simulink model "CM640A_MotAg1Meas"  (R2013b)
settings: Solver=FixedStepDiscrete  SolverMode=SingleTasking  StartTime=0.0  StopTime=1  FixedStep=0.0000625  RelTol=1e-3
undefined symbols (not defined in the file): ARCHGLBPRM_2PI_ULS_F32, COEFFTBLELMSIZE_CNT_U08, COEFFTBLSIZE_CNT_U08, CORRNTBLAGSTEPSIZE_MATRAD_F32, CORRNTBLSIDXOFFS_CNT_U16, CORRNTBLSIZE_CNT_U16, CORRNTBLSIZEMASK_CNT_U08, MOTAG1OFFS_MOTREV_U0P16, MotAg1PrtclFlt, MOTAG1PRTCLFLTFAILSTEP_CNT_U16, MOTAG1PRTCLFLTPASSSTEP_CNT_U16, MOTAGDELTAPERCORRNPT_CNT_U16, MOTAGIDXMASK_CNT_U16, MotCtrlMotAg1ErrReg, NtcSts1, sigbuilder_block, SNSRAGMASK_CNT_U32, SNSRERRMASK_CNT_U32, SNSRERRNTCMASK_CNT_U08, SNSRVLTGFLTMASK_CNT_U32, SPIPARMASK_CNT_U32
libraries: simulink x28, FloatToFixd x1, NxtrMax x1, NxtrLim x1
(part 2 of 4)

== system CM640A_MotAg1Meas/MotAg1Meas/MotAg1MeasPer2/Process ErrorReg and DieRevCtr ==
  MotAg1ErrReg : Inport  OutDataTypeStr=uint32
  CopyRight2 : Subsystem  Description=|  mask(Copyright Information){none=on}
      | Copyright info block.                                               
      |                                                                     
      | Place copyright information at the top of every subsystem in design.
      mask prompts: none "No parameters"
      mask help: Place copyright information at the top of every subsystem in design.
      mask Display:
      | NxtrConf = 'Nexteer Confidential';
      | 
      | sys = bdroot; %handle for the current model ("system")
      | first = get_param(sys,'Created');
      | first = first(end-3:end);  %year is last four digits
      | 
      | last = get_param(sys,'LastModifiedDate');
      | if isempty(last)
      |     last = datestr(now,'yyyy');
      | else
      |     last = last(end-3:end);
      | end
      | 
      | if strcmp(first,last)
      |     fprintf('%s -- Copyright %s Nexteer',NxtrConf,first)
      | else
      |     fprintf('%s -- %s%s- %s Nexteer',NxtrConf,char(169),first,last)
      | end
  Process MotAg1RawErr : Subsystem  RequirementInfo={} %GIDa_05fef35d_e67f_443b_a4d0_6048385f8050
  MotAg1Err : Outport  OutDataTypeStr=uint8
  MotAg1ErrParFltCnt : Outport  Port=2
  wires:
  MotAg1ErrReg/1 -> Process MotAg1RawErr/1(MotAg1ErrReg)
  Process MotAg1RawErr/1(MotAg1ErrParFltCnt) -> MotAg1ErrParFltCnt/1
  Process MotAg1RawErr/2(MotAg1Err) -> MotAg1Err/1

== system CM640A_MotAg1Meas/MotAg1Meas/MotAg1MeasInit1/Compute Correction Table/CopyRight2 ==

== system CM640A_MotAg1Meas/MotAg1Meas/MotAg1MeasInit1/Compute Correction Table/MotAg1CorrnTbl_GetErrorStatus ==
  note: 0 simulated for modeling purposes,
      | actual value returned by NVM.  Non-zero return indicates
      | failure in storage/retrievial of NVM.
  Constant : Constant  Value=0
  CopyRight2 : Subsystem  Description=|  mask(Copyright Information){none=on}
      | Copyright info block.                                               
      |                                                                     
      | Place copyright information at the top of every subsystem in design.
      mask prompts: none "No parameters"
      mask help: Place copyright information at the top of every subsystem in design.
      mask Display:
      | NxtrConf = 'Nexteer Confidential';
      | 
      | sys = bdroot; %handle for the current model ("system")
      | first = get_param(sys,'Created');
      | first = first(end-3:end);  %year is last four digits
      | 
      | last = get_param(sys,'LastModifiedDate');
      | if isempty(last)
      |     last = datestr(now,'yyyy');
      | else
      |     last = last(end-3:end);
      | end
      | 
      | if strcmp(first,last)
      |     fprintf('%s -- Copyright %s Nexteer',NxtrConf,first)
      | else
      |     fprintf('%s -- %s%s- %s Nexteer',NxtrConf,char(169),first,last)
      | end
  RequestResultPtr : Outport
  wires:
  Constant/1 -> RequestResultPtr/1

== system CM640A_MotAg1Meas/MotAg1Meas/MotAg1MeasInit1/Compute Correction Table/NVM NOK ==
  note: In the event of a NVM failure
      | set the correction table to 0
  Action Port : ActionPort  ActionType=else
  Constant1 : Constant  Value=CORRNTBLSIZE_CNT_U16
  CopyRight2 : Subsystem  Description=|  mask(Copyright Information){none=on}
      | Copyright info block.                                               
      |                                                                     
      | Place copyright information at the top of every subsystem in design.
      mask prompts: none "No parameters"
      mask help: Place copyright information at the top of every subsystem in design.
      mask Display:
      | NxtrConf = 'Nexteer Confidential';
      | 
      | sys = bdroot; %handle for the current model ("system")
      | first = get_param(sys,'Created');
      | first = first(end-3:end);  %year is last four digits
      | 
      | last = get_param(sys,'LastModifiedDate');
      | if isempty(last)
      |     last = datestr(now,'yyyy');
      | else
      |     last = last(end-3:end);
      | end
      | 
      | if strcmp(first,last)
      |     fprintf('%s -- Copyright %s Nexteer',NxtrConf,first)
      | else
      |     fprintf('%s -- %s%s- %s Nexteer',NxtrConf,char(169),first,last)
      | end
  Zero out correction table : Subsystem  TreatAsAtomicUnit=on
  wires:
  Constant1/1 -> Zero out correction table/1(N)

== system CM640A_MotAg1Meas/MotAg1Meas/MotAg1MeasInit1/Compute Correction Table/NVM Ok ==
  Action Port : ActionPort  ActionType=then
  Calculate Correction Table : Subsystem  Priority=100  TreatAsAtomicUnit=on
      settings: AttributesFormatString=|
      | Priority:
      | %<Priority>
  Configure Coefficients : Subsystem  Priority=10  TreatAsAtomicUnit=on
      settings: AttributesFormatString=|
      | Priority:
      | %<Priority>
  CopyRight2 : Subsystem  Description=|  mask(Copyright Information){none=on}
      | Copyright info block.                                               
      |                                                                     
      | Place copyright information at the top of every subsystem in design.
      mask prompts: none "No parameters"
      mask help: Place copyright information at the top of every subsystem in design.
      mask Display:
      | NxtrConf = 'Nexteer Confidential';
      | 
      | sys = bdroot; %handle for the current model ("system")
      | first = get_param(sys,'Created');
      | first = first(end-3:end);  %year is last four digits
      | 
      | last = get_param(sys,'LastModifiedDate');
      | if isempty(last)
      |     last = datestr(now,'yyyy');
      | else
      |     last = last(end-3:end);
      | end
      | 
      | if strcmp(first,last)
      |     fprintf('%s -- Copyright %s Nexteer',NxtrConf,first)
      | else
      |     fprintf('%s -- %s%s- %s Nexteer',NxtrConf,char(169),first,last)
      | end

== system CM640A_MotAg1Meas/MotAg1Meas/MotAg1MeasInit1/Initialize CSIH RAM1/CopyRight2 ==

== system CM640A_MotAg1Meas/MotAg1Meas/MotAg1MeasPer1/Compensate MechMtrPos/CopyRight1 ==

== system CM640A_MotAg1Meas/MotAg1Meas/MotAg1MeasPer1/Process MotAg1 Angle/CopyRight2 ==

== system CM640A_MotAg1Meas/MotAg1Meas/MotAg1MeasPer1/Process MotAg1 Angle/Process MotAg1Raw ==
  RxMtrPosReg_Cnt_u32 : Inport  OutDataTypeStr=uint32
  CopyRight2 : Subsystem  Description=|  mask(Copyright Information){none=on}
      | Copyright info block.                                               
      |                                                                     
      | Place copyright information at the top of every subsystem in design.
      mask prompts: none "No parameters"
      mask help: Place copyright information at the top of every subsystem in design.
      mask Display:
      | NxtrConf = 'Nexteer Confidential';
      | 
      | sys = bdroot; %handle for the current model ("system")
      | first = get_param(sys,'Created');
      | first = first(end-3:end);  %year is last four digits
      | 
      | last = get_param(sys,'LastModifiedDate');
      | if isempty(last)
      |     last = datestr(now,'yyyy');
      | else
      |     last = last(end-3:end);
      | end
      | 
      | if strcmp(first,last)
      |     fprintf('%s -- Copyright %s Nexteer',NxtrConf,first)
      | else
      |     fprintf('%s -- %s%s- %s Nexteer',NxtrConf,char(169),first,last)
      | end
  MotAg Message Parity Monitoring : Subsystem  RequirementInfo="{'linktype_rmi_doors' '0000cf48 (/ESG Group/FDD Module Requirements/EA4 Specific/CM640A_MotAg1Meas)' '#CM640A_93' 'true' 'REQ:  CM640A_93' '' } %GIDa_0575b366_3fb8_4b54_8653_e88c552f3ea4"  TreatAsAtomicUnit=on
  Raw Mecl Mot Ag Processing : Subsystem  RequirementInfo="{'linktype_rmi_doors' '0000cf48 (/ESG Group/FDD Module Requirements/EA4 Specific/CM640A_MotAg1Meas)' '#CM640A_84' 'true' 'REQ:  CM640A_84' '' } %GIDa_bdb55e65_3f35_4b3c_b59f_3789084d0974"  TreatAsAtomicUnit=on
  Undervoltage Bit Monitoring : Subsystem  RequirementInfo="{'linktype_rmi_doors' '0000cf48 (/ESG Group/FDD Module Requirements/EA4 Specific/CM640A_MotAg1Meas)' '#CM640A_86' 'true' 'REQ:  CM640A_86' '' } %GIDa_7bdb6e2d_fd76_45a7_a9c7_b8b57ac688de"  TreatAsAtomicUnit=on
  MotAg1VltgFlt : Outport
  MotAg1ParFlt : Outport  Port=2
  MotAg1RawMecl : Outport  Port=3
  wires:
  RxMtrPosReg_Cnt_u32/1 -> Raw Mecl Mot Ag Processing/1(RxMtrPosReg_Cnt_u32), MotAg Message Parity Monitoring/1(RxMtrPosReg_Cnt_u32), Undervoltage Bit Monitoring/1(RxMtrPosReg_Cnt_u32)
  Raw Mecl Mot Ag Processing/1(MotAg1RawMecl) -> MotAg1RawMecl/1
  Undervoltage Bit Monitoring/1(MotAg1VltgFlt) -> MotAg1VltgFlt/1
  MotAg Message Parity Monitoring/1(MotAg1ParFlt) -> MotAg1ParFlt/1

== system CM640A_MotAg1Meas/MotAg1Meas/MotAg1MeasPer1/Process MotAg1 Angle/Protocol Present Handling ==
  Protocol Fault Present : Inport
  MotAg1RawMecl Input : Inport  Port=2
  CopyRight2 : Subsystem  Description=|  mask(Copyright Information){none=on}
      | Copyright info block.                                               
      |                                                                     
      | Place copyright information at the top of every subsystem in design.
      mask prompts: none "No parameters"
      mask help: Place copyright information at the top of every subsystem in design.
      mask Display:
      | NxtrConf = 'Nexteer Confidential';
      | 
      | sys = bdroot; %handle for the current model ("system")
      | first = get_param(sys,'Created');
      | first = first(end-3:end);  %year is last four digits
      | 
      | last = get_param(sys,'LastModifiedDate');
      | if isempty(last)
      |     last = datestr(now,'yyyy');
      | else
      |     last = last(end-3:end);
      | end
      | 
      | if strcmp(first,last)
      |     fprintf('%s -- Copyright %s Nexteer',NxtrConf,first)
      | else
      |     fprintf('%s -- %s%s- %s Nexteer',NxtrConf,char(169),first,last)
      | end
  If : If  IfExpression=u1 == 0
  "Invalid Polarity, Hold Last Value" : Subsystem  TreatAsAtomicUnit=on
  Merge : Merge  RequirementInfo={} %GIDa_c39e7a9a_c902_423e_a1fe_e344504ccac1
  Unit Delay3 : UnitDelay  SampleTime=-1  StateName=MotAg1RawMeclPrev  StateMustResolveToSignalObject=on
      settings: AttributesFormatString=|
      | State Variable:
      | %<StateName>
  Valid Polarity : Subsystem  TreatAsAtomicUnit=on
  MotAg1RawMecl : Outport
  wires:
  Unit Delay3/1 -> "Invalid Polarity, Hold Last Value"/1(In1)
  Merge/1 -> MotAg1RawMecl/1, Unit Delay3/1
  "Invalid Polarity, Hold Last Value"/1(Out1) -> Merge/2
  Valid Polarity/1(Out1) -> Merge/1
  If/2 -> "Invalid Polarity, Hold Last Value"/Action
  If/1 -> Valid Polarity/Action
  MotAg1RawMecl Input/1 -> Valid Polarity/1(In1)
  Protocol Fault Present/1 -> If/1

== system CM640A_MotAg1Meas/MotAg1Meas/MotAg1MeasPer2/MotAg1 Protocol Fault Operation/Atomic Subsystem ==
  NtcStInfo : Inport  OutDataTypeStr=uint8
  CopyRight2 : Subsystem  Description=|  mask(Copyright Information){none=on}
      | Copyright info block.                                               
      |                                                                     
      | Place copyright information at the top of every subsystem in design.
      mask prompts: none "No parameters"
      mask help: Place copyright information at the top of every subsystem in design.
      mask Display:
      | NxtrConf = 'Nexteer Confidential';
      | 
      | sys = bdroot; %handle for the current model ("system")
      | first = get_param(sys,'Created');
      | first = first(end-3:end);  %year is last four digits
      | 
      | last = get_param(sys,'LastModifiedDate');
      | if isempty(last)
      |     last = datestr(now,'yyyy');
      | else
      |     last = last(end-3:end);
      | end
      | 
      | if strcmp(first,last)
      |     fprintf('%s -- Copyright %s Nexteer',NxtrConf,first)
      | else
      |     fprintf('%s -- %s%s- %s Nexteer',NxtrConf,char(169),first,last)
      | end
  If : If
  Merge : Merge
  Merge1 : Merge
  N Step : Subsystem  RequirementInfo="{'linktype_rmi_doors' '0000cf48 (/ESG Group/FDD Module Requirements/EA4 Specific/CM640A_MotAg1Meas)' '#CM640A_31' 'true' 'REQ:  CM640A_31' '' } %GIDa_a1ed8da0_4c35_4cb0_a2c6_08587c652881"  TreatAsAtomicUnit=on
  P Step : Subsystem  TreatAsAtomicUnit=on
  NtcSts : Outport
  DebStep : Outport  Port=2  OutDataTypeStr=uint16
  wires:
  NtcStInfo/1 -> If/1
  If/1 -> P Step/Action
  If/2 -> N Step/Action
  Merge/1 -> DebStep/1
  P Step/1(NtcSts) -> Merge1/1
  N Step/1(NtcSts) -> Merge1/2
  Merge1/1 -> NtcSts/1
  P Step/2(DebStep) -> Merge/1
  N Step/2(DebStep) -> Merge/2

== system CM640A_MotAg1Meas/MotAg1Meas/MotAg1MeasPer2/MotAg1 Protocol Fault Operation/CopyRight2 ==

== system CM640A_MotAg1Meas/MotAg1Meas/MotAg1MeasPer2/MotAg1 Protocol Fault Operation/GetNtcQlfr ==
  NtcNr : Inport
  CopyRight2 : Subsystem  Description=|  mask(Copyright Information){none=on}
      | Copyright info block.                                               
      |                                                                     
      | Place copyright information at the top of every subsystem in design.
      mask prompts: none "No parameters"
      mask help: Place copyright information at the top of every subsystem in design.
      mask Display:
      | NxtrConf = 'Nexteer Confidential';
      | 
      | sys = bdroot; %handle for the current model ("system")
      | first = get_param(sys,'Created');
      | first = first(end-3:end);  %year is last four digits
      | 
      | last = get_param(sys,'LastModifiedDate');
      | if isempty(last)
      |     last = datestr(now,'yyyy');
      | else
      |     last = last(end-3:end);
      | end
      | 
      | if strcmp(first,last)
      |     fprintf('%s -- Copyright %s Nexteer',NxtrConf,first)
      | else
      |     fprintf('%s -- %s%s- %s Nexteer',NxtrConf,char(169),first,last)
      | end
  Data Store Read : DataStoreRead  DataStoreName=NtcQlfr
  Terminator : Terminator
  NtcQlfr : Outport
  wires:
  NtcNr/1 -> Terminator/1
  Data Store Read/1 -> NtcQlfr/1

== system CM640A_MotAg1Meas/MotAg1Meas/MotAg1MeasPer2/MotAg1 Protocol Fault Operation/SetNtcSts ==
  note: Note:
      |
      | - "ISO Fault Debounce Design" Simulink block intent to use here for Simulation purpose only. Do not Code this block
  NtcNr : Inport
  NtcStInfo : Inport  Port=2
  NtcSts : Inport  Port=3  OutDataTypeStr=Enum: NtcSts1
  DebStep : Inport  Port=4
  CopyRight2 : Subsystem  Description=|  mask(Copyright Information){none=on}
      | Copyright info block.                                               
      |                                                                     
      | Place copyright information at the top of every subsystem in design.
      mask prompts: none "No parameters"
      mask help: Place copyright information at the top of every subsystem in design.
      mask Display:
      | NxtrConf = 'Nexteer Confidential';
      | 
      | sys = bdroot; %handle for the current model ("system")
      | first = get_param(sys,'Created');
      | first = first(end-3:end);  %year is last four digits
      | 
      | last = get_param(sys,'LastModifiedDate');
      | if isempty(last)
      |     last = datestr(now,'yyyy');
      | else
      |     last = last(end-3:end);
      | end
      | 
      | if strcmp(first,last)
      |     fprintf('%s -- Copyright %s Nexteer',NxtrConf,first)
      | else
      |     fprintf('%s -- %s%s- %s Nexteer',NxtrConf,char(169),first,last)
      | end
  Data Store Write : DataStoreWrite  DataStoreName=NtcQlfr
  Data Type Conversion1 : DataTypeConversion  OutDataTypeStr=uint8
  Ground : Ground
  ISO Fault Debounce Design : Stateflow chart  TreatAsAtomicUnit=on
      settings: AttributesFormatString=|
      | Simulation Purpose Only.
      | Do Not Code this block
      | Diagnostic Manager Owns this requirement
  Scope1 : Scope  NumInputPorts=4
      settings: YMin=-5~-5~-5~-5  YMax=5~5~5~5  SaveName=ScopeData5
  Terminator : Terminator
  Terminator1 : Terminator
  wires:
  NtcStInfo/1 -> Scope1/4, Terminator1/1
  NtcNr/1 -> Terminator/1
  NtcSts/1 -> Data Type Conversion1/1
  DebStep/1 -> ISO Fault Debounce Design/2(DebStep), Scope1/2
  ISO Fault Debounce Design/1(Qualifier) -> Scope1/3, Data Store Write/1
  Ground/1 -> ISO Fault Debounce Design/3(SvcClr)
  Data Type Conversion1/1 -> ISO Fault Debounce Design/1(NtcSts), Scope1/1

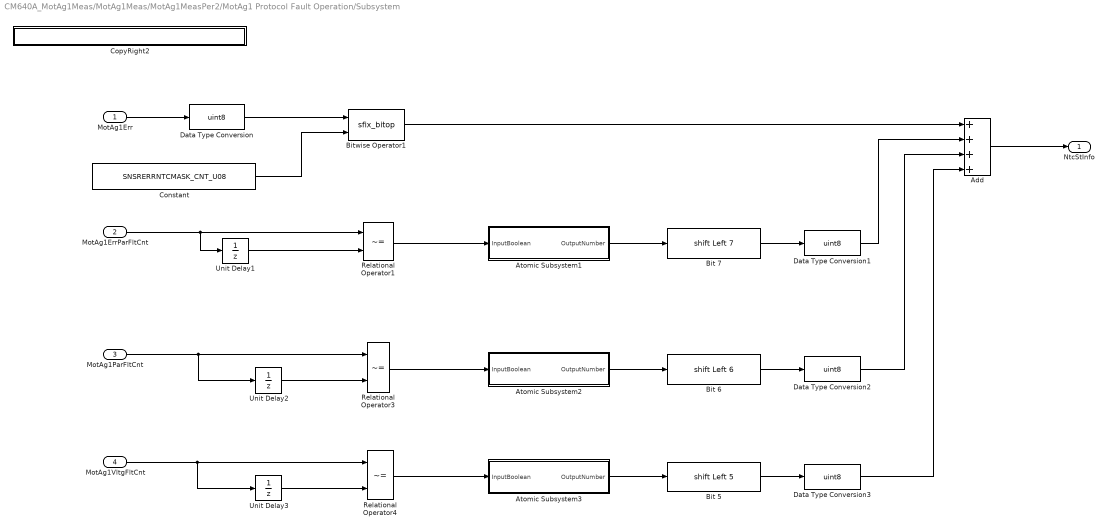
== system CM640A_MotAg1Meas/MotAg1Meas/MotAg1MeasPer2/MotAg1 Protocol Fault Operation/Subsystem ==
  MotAg1Err : Inport  RequirementInfo={} %GIDa_6edd1ae9_9c74_4544_bf40_7d9417b836a7
  MotAg1ErrParFltCnt : Inport  Port=2
  MotAg1ParFltCnt : Inport  Port=3
  MotAg1VltgFltCnt : Inport  Port=4
  Add : Sum  Inputs=++++
  Atomic Subsystem1 : Subsystem  TreatAsAtomicUnit=on
  Atomic Subsystem2 : Subsystem  TreatAsAtomicUnit=on
  Atomic Subsystem3 : Subsystem  TreatAsAtomicUnit=on
  Bit 5 : ArithShift  RequirementInfo="{'linktype_rmi_doors' '0000cf48 (/ESG Group/FDD Module Requirements/EA4 Specific/CM640A_MotAg1Meas)' '#CM640A_28' 'true' 'REQ:  CM640A_28' '' } %GIDa_baaec4dd_391c_4963_979e_8a787ae9f4f7"  BitShiftNumber=5  BitShiftDirection=Left
  Bit 6 : ArithShift  RequirementInfo="{'linktype_rmi_doors' '0000cf48 (/ESG Group/FDD Module Requirements/EA4 Specific/CM640A_MotAg1Meas)' '#CM640A_101' 'true' 'REQ:  CM640A_101' '' } %GIDa_688756ca_05b1_4787_ba54_8f8dae8f5212"  BitShiftNumber=6  BitShiftDirection=Left
  Bit 7 : ArithShift  RequirementInfo="{'linktype_rmi_doors' '0000cf48 (/ESG Group/FDD Module Requirements/EA4 Specific/CM640A_MotAg1Meas)' '#CM640A_102' 'true' 'REQ:  CM640A_102' '' } %GIDa_5f89c88f_2af9_4850_b51d_5320054dccdc"  BitShiftNumber=7  BitShiftDirection=Left
  Bitwise Operator1 : S-Function  RequirementInfo="{'linktype_rmi_doors' '0000cf48 (/ESG Group/FDD Module Requirements/EA4 Specific/CM640A_MotAg1Meas)' '#CM640A_91' 'true' 'REQ:  CM640A_91' '' ; 'linktype_rmi_doors' '0000cf48 (/ESG Group/FDD Module Requirements/EA4 Specific/CM640A_MotAg1Meas)' '#CM640A_98' 'true' 'REQ:  CM640A_98' '' ; 'linktype_rmi_doors' '0000cf48 (/ESG Group/FDD Module Requirements/EA4 Specific/CM640A_MotAg1Meas)' '#CM640A_99' 'true' 'REQ:  CM640A_99' '' ; 'linktype_rmi_doors' '0000cf48 (/ESG Group/FDD Module Requirements/EA4 Specific/CM640A_MotAg1Meas)' '#CM640A_100' 'true' 'REQ:  CM640A_100' '' } %GIDa_5c9d0cb2_6ffb_4aa7_875c_2abe2058166d"  FunctionName=sfix_bitop  Parameters=UseBitMask,NumInputPorts,BitMask,BitMaskRealWorld,logicop  EnableBusSupport=off  mask(Bitwise Operator){logicop=AND, UseBitMask=off, NumInputPorts=2, BitMask=SNSRERRNTCMASK_CNT_U08, BitMaskRealWorld=Stored Integer}
      mask prompts: logicop "Operator:"; UseBitMask "Use bit mask ..."; NumInputPorts "Number of input ports:"; BitMask "Bit Mask"; BitMaskRealWorld "Treat mask as:"
      mask help: Perform the specified bitwise operation on the inputs. The output data type should represent zero exactly.
      mask init:
      | str = '';
      | if UseBitMask
      |   [m,n] = size(BitMask);
      |   if ischar(BitMask)
      |     len = m;
      |     n = 1;
      |   else
      |     len = m * n;
      |   end
      |   internalBitMask = zeros(m,n);
      |   if isnumeric(BitMask)
      |     for i=1:len,
      |       internalBitMask(i) = BitMask(i);
      |     end
      |   elseif ischar(BitMask)
      |     for i=1:m,
      |       internalBitMask(i) = hex2dec(BitMask(i,:));
      |     end
      |   elseif iscell(BitMask)
      |     for i=1:len,
      |       if isnumeric( BitMask{i} )
      |         internalBitMask(i) = BitMask{i};
      |       elseif ischar( BitMask{i} )
      |         internalBitMask(i) = hex2dec(BitMask{i});
      |       else
      |         errordlg(['Data type is not supported at cell item ', num2str(i) ]);
      |       end
      |     end
      |   end
      |   BitMask = internalBitMask;
      |   for i=1:len
      |     if BitMask(i) > (2^52)-1
      |       error(DAStudio.message('Simulink:blocks:BitMaskWordLengthTooLarge')); 
      |     end
      |   end 
      |   if len == 1
      |      if BitMaskRealWorld == 1 || BitMask(1) < 0
      |        str=num2str(BitMask(1));
      |      else
      |        str=['0x',dec2hex(floor(BitMask(1)))];
      |      end
      |   else
      |      str='Masks';
      |   end
      | else
      |   BitMask = 0;
      |   str='';
      | end
      mask TypeOptions logicop: AND | OR | NAND | NOR | XOR | NOT
      mask Callback logicop: fixptdialog(gcbh)
      mask Callback UseBitMask: fixptdialog(gcbh)
      mask TypeOptions BitMaskRealWorld: Real World Value | Stored Integer
      mask Display: fprintf(['Bitwise\n',logicop,'\n',str])
  Constant : Constant  Value=SNSRERRNTCMASK_CNT_U08
  CopyRight2 : Subsystem  Description=|  mask(Copyright Information){none=on}
      | Copyright info block.                                               
      |                                                                     
      | Place copyright information at the top of every subsystem in design.
      mask prompts: none "No parameters"
      mask help: Place copyright information at the top of every subsystem in design.
      mask Display:
      | NxtrConf = 'Nexteer Confidential';
      | 
      | sys = bdroot; %handle for the current model ("system")
      | first = get_param(sys,'Created');
      | first = first(end-3:end);  %year is last four digits
      | 
      | last = get_param(sys,'LastModifiedDate');
      | if isempty(last)
      |     last = datestr(now,'yyyy');
      | else
      |     last = last(end-3:end);
      | end
      | 
      | if strcmp(first,last)
      |     fprintf('%s -- Copyright %s Nexteer',NxtrConf,first)
      | else
      |     fprintf('%s -- %s%s- %s Nexteer',NxtrConf,char(169),first,last)
      | end
  Data Type Conversion{,1..3} (4 alike) : DataTypeConversion  OutDataTypeStr=uint8
  Relational Operator1 : RelationalOperator  Operator=~=  OutDataTypeStr=boolean
  Relational Operator3 : RelationalOperator  Operator=~=  OutDataTypeStr=boolean
  Relational Operator4 : RelationalOperator  Operator=~=  OutDataTypeStr=boolean
  Unit Delay1 : UnitDelay  SampleTime=-1  StateName=MotAg1ErrParFltNtcStInfoCntPrev  StateMustResolveToSignalObject=on
      settings: AttributesFormatString=|
      | State Variable:
      | %<StateName>
  Unit Delay2 : UnitDelay  SampleTime=-1  StateName=MotAg1ParFltNtcStInfoCntPrev  StateMustResolveToSignalObject=on
      settings: AttributesFormatString=|
      | State Variable:
      | %<StateName>
  Unit Delay3 : UnitDelay  SampleTime=-1  StateName=MotAg1VltgFltNtcStInfoCntPrev  StateMustResolveToSignalObject=on
      settings: AttributesFormatString=|
      | State Variable:
      | %<StateName>
  NtcStInfo : Outport
  wires:
  Add/1 -> NtcStInfo/1
  Relational Operator3/1 -> Atomic Subsystem2/1(InputBoolean)
  MotAg1ParFltCnt/1 -> Unit Delay2/1, Relational Operator3/1
  Unit Delay1/1 -> Relational Operator1/2
  MotAg1ErrParFltCnt/1 -> Unit Delay1/1, Relational Operator1/1
  MotAg1Err/1 -> Data Type Conversion/1
  Data Type Conversion/1 -> Bitwise Operator1/1
  Relational Operator4/1 -> Atomic Subsystem3/1(InputBoolean)
  Unit Delay3/1 -> Relational Operator4/2
  MotAg1VltgFltCnt/1 -> Unit Delay3/1, Relational Operator4/1
  Bitwise Operator1/1 -> Add/1
  Unit Delay2/1 -> Relational Operator3/2
  Relational Operator1/1 -> Atomic Subsystem1/1(InputBoolean)
  Atomic Subsystem1/1(OutputNumber) -> Bit 7/1
  Atomic Subsystem2/1(OutputNumber) -> Bit 6/1
  Atomic Subsystem3/1(OutputNumber) -> Bit 5/1
  Data Type Conversion3/1 -> Add/4
  Data Type Conversion2/1 -> Add/3
  Data Type Conversion1/1 -> Add/2
  Bit 5/1 -> Data Type Conversion3/1
  Bit 6/1 -> Data Type Conversion2/1
  Bit 7/1 -> Data Type Conversion1/1
  Constant/1 -> Bitwise Operator1/2

== system CM640A_MotAg1Meas/MotAg1Meas/MotAg1MeasPer2/Process ErrorReg and DieRevCtr/CopyRight2 ==

== system CM640A_MotAg1Meas/MotAg1Meas/MotAg1MeasPer2/Process ErrorReg and DieRevCtr/Process MotAg1RawErr ==
  MotAg1ErrReg : Inport
  Chart1 : Stateflow chart  TreatAsAtomicUnit=on
  CopyRight2 : Subsystem  Description=|  mask(Copyright Information){none=on}
      | Copyright info block.                                               
      |                                                                     
      | Place copyright information at the top of every subsystem in design.
      mask prompts: none "No parameters"
      mask help: Place copyright information at the top of every subsystem in design.
      mask Display:
      | NxtrConf = 'Nexteer Confidential';
      | 
      | sys = bdroot; %handle for the current model ("system")
      | first = get_param(sys,'Created');
      | first = first(end-3:end);  %year is last four digits
      | 
      | last = get_param(sys,'LastModifiedDate');
      | if isempty(last)
      |     last = datestr(now,'yyyy');
      | else
      |     last = last(end-3:end);
      | end
      | 
      | if strcmp(first,last)
      |     fprintf('%s -- Copyright %s Nexteer',NxtrConf,first)
      | else
      |     fprintf('%s -- %s%s- %s Nexteer',NxtrConf,char(169),first,last)
      | end
  Data Type Conversion1 : DataTypeConversion  OutDataTypeStr=uint16
  If : If  IfExpression=u1 == 0
  "Invalid Polarity, Hold Last Value" : Subsystem  TreatAsAtomicUnit=on
  Merge : Merge
  Process MotAg1RawErr : Subsystem
  Unit Delay1 : UnitDelay  SampleTime=-1  StateName=MotAg1ErrParFltCntPrev  StateMustResolveToSignalObject=on
      settings: AttributesFormatString=|
      | State Variable:
      | %<StateName>
  Unit Delay3 : UnitDelay  SampleTime=-1  StateName=MotAg1ErrPrev  StateMustResolveToSignalObject=on
      settings: AttributesFormatString=|
      | State Variable:
      | %<StateName>
  Valid Polarity : Subsystem  TreatAsAtomicUnit=on
  MotAg1ErrParFltCnt : Outport
  MotAg1Err : Outport  Port=2  OutDataTypeStr=uint8
  wires:
  Process MotAg1RawErr/1(MotAg1ErrParFlt) -> If/1, Data Type Conversion1/1
  Unit Delay3/1 -> "Invalid Polarity, Hold Last Value"/1(In1)
  Merge/1 -> Unit Delay3/1, MotAg1Err/1
  MotAg1ErrReg/1 -> Process MotAg1RawErr/1(MotAg1ErrReg)
  "Invalid Polarity, Hold Last Value"/1(Out1) -> Merge/2
  Valid Polarity/1(Out1) -> Merge/1
  If/2 -> "Invalid Polarity, Hold Last Value"/Action
  If/1 -> Valid Polarity/Action
  Process MotAg1RawErr/2(MotAg1Err) -> Valid Polarity/1(In1)
  Data Type Conversion1/1 -> Chart1/1(Fault)
  Chart1/1(FaultCnt) -> MotAg1ErrParFltCnt/1, Unit Delay1/1
  Unit Delay1/1 -> Chart1/2(FaultCntPrev)

== system CM640A_MotAg1Meas/MotAg1Meas/MotAg1MeasInit1/Compute Correction Table/MotAg1CorrnTbl_GetErrorStatus/CopyRight2 ==

== system CM640A_MotAg1Meas/MotAg1Meas/MotAg1MeasInit1/Compute Correction Table/NVM NOK/CopyRight2 ==

== system CM640A_MotAg1Meas/MotAg1Meas/MotAg1MeasInit1/Compute Correction Table/NVM NOK/Zero out correction table ==
  N : Inport
  Assignment : Assignment  IndexMode=Zero-based  IndexOptions=Index vector (port)  Indices=1  OutputSizes=1
  CopyRight2 : Subsystem  Description=|  mask(Copyright Information){none=on}
      | Copyright info block.                                               
      |                                                                     
      | Place copyright information at the top of every subsystem in design.
      mask prompts: none "No parameters"
      mask help: Place copyright information at the top of every subsystem in design.
      mask Display:
      | NxtrConf = 'Nexteer Confidential';
      | 
      | sys = bdroot; %handle for the current model ("system")
      | first = get_param(sys,'Created');
      | first = first(end-3:end);  %year is last four digits
      | 
      | last = get_param(sys,'LastModifiedDate');
      | if isempty(last)
      |     last = datestr(now,'yyyy');
      | else
      |     last = last(end-3:end);
      | end
      | 
      | if strcmp(first,last)
      |     fprintf('%s -- Copyright %s Nexteer',NxtrConf,first)
      | else
      |     fprintf('%s -- %s%s- %s Nexteer',NxtrConf,char(169),first,last)
      | end
  Data Store Read : DataStoreRead  DataStoreName=MotAg1CorrnTbl
  Data Store Write : DataStoreWrite  DataStoreName=MotAg1CorrnTbl
  For Iterator : ForIterator  ResetStates=reset  IterationSource=external  IndexMode=Zero-based  IterationVariableDataType=int16
  Zero : Constant  Value=0  OutDataTypeStr=int8
  wires:
  For Iterator/1 -> Assignment/3
  N/1 -> For Iterator/1
  Data Store Read/1 -> Assignment/1
  Assignment/1 -> Data Store Write/1
  Zero/1 -> Assignment/2

== system CM640A_MotAg1Meas/MotAg1Meas/MotAg1MeasInit1/Compute Correction Table/NVM Ok/Calculate Correction Table ==
  Build Wave : Subsystem  RequirementInfo="{'linktype_rmi_doors' '0000cf48 (/ESG Group/FDD Module Requirements/EA4 Specific/CM640A_MotAg1Meas)' '#CM640A_118' 'true' 'REQ:  CM640A_118' '' } %GIDa_a6dafb17_ad26_4c6e_b476_48d6decc7b31"  TreatAsAtomicUnit=on
  Change Correction Coordinate : Subsystem  RequirementInfo="{'linktype_rmi_doors' '0000cf48 (/ESG Group/FDD Module Requirements/EA4 Specific/CM640A_MotAg1Meas)' '#CM640A_119' 'true' 'REQ:  CM640A_119' '' } %GIDa_ff21555f_fb16_4d1c_92dc_4427cf6bec33"  TreatAsAtomicUnit=on
  CopyRight2 : Subsystem  Description=|  mask(Copyright Information){none=on}
      | Copyright info block.                                               
      |                                                                     
      | Place copyright information at the top of every subsystem in design.
      mask prompts: none "No parameters"
      mask help: Place copyright information at the top of every subsystem in design.
      mask Display:
      | NxtrConf = 'Nexteer Confidential';
      | 
      | sys = bdroot; %handle for the current model ("system")
      | first = get_param(sys,'Created');
      | first = first(end-3:end);  %year is last four digits
      | 
      | last = get_param(sys,'LastModifiedDate');
      | if isempty(last)
      |     last = datestr(now,'yyyy');
      | else
      |     last = last(end-3:end);
      | end
      | 
      | if strcmp(first,last)
      |     fprintf('%s -- Copyright %s Nexteer',NxtrConf,first)
      | else
      |     fprintf('%s -- %s%s- %s Nexteer',NxtrConf,char(169),first,last)
      | end

== system CM640A_MotAg1Meas/MotAg1Meas/MotAg1MeasInit1/Compute Correction Table/NVM Ok/Configure Coefficients ==
  note: This block is for simulation purposes only.
      |
      | The data in shadowed RAM is to be populated
      | by NVM handler
  CopyRight2 : Subsystem  Description=|  mask(Copyright Information){none=on}
      | Copyright info block.                                               
      |                                                                     
      | Place copyright information at the top of every subsystem in design.
      mask prompts: none "No parameters"
      mask help: Place copyright information at the top of every subsystem in design.
      mask Display:
      | NxtrConf = 'Nexteer Confidential';
      | 
      | sys = bdroot; %handle for the current model ("system")
      | first = get_param(sys,'Created');
      | first = first(end-3:end);  %year is last four digits
      | 
      | last = get_param(sys,'LastModifiedDate');
      | if isempty(last)
      |     last = datestr(now,'yyyy');
      | else
      |     last = last(end-3:end);
      | end
      | 
      | if strcmp(first,last)
      |     fprintf('%s -- Copyright %s Nexteer',NxtrConf,first)
      | else
      |     fprintf('%s -- %s%s- %s Nexteer',NxtrConf,char(169),first,last)
      | end
  Data Store Write : DataStoreWrite  DataStoreName=MotAg1CoeffTbl
  temporary harmonic coefficient holder : Constant  Value=[0 0 0.0199999995529651642 0 0 0 0 0 0 0 0 0 0 0 0 0 0 0 0 0 0 0 0 0 0 0]  OutDataTypeStr=single
  wires:
  temporary harmonic coefficient holder/1 -> Data Store Write/1

== system CM640A_MotAg1Meas/MotAg1Meas/MotAg1MeasInit1/Compute Correction Table/NVM Ok/CopyRight2 ==

== system CM640A_MotAg1Meas/MotAg1Meas/MotAg1MeasPer1/Process MotAg1 Angle/Process MotAg1Raw/CopyRight2 ==

== system CM640A_MotAg1Meas/MotAg1Meas/MotAg1MeasPer1/Process MotAg1 Angle/Process MotAg1Raw/MotAg Message Parity Monitoring ==
  RxMtrPosReg_Cnt_u32 : Inport
  Atomic Subsystem2 : Subsystem  TreatAsAtomicUnit=on
  Atomic Subsystem3 : Subsystem  TreatAsAtomicUnit=on
  Bitwise Operator3 : simulink/Logic and Bit Operations/Bitwise Operator  logicop=AND  UseBitMask=off  NumInputPorts=2  BitMask=SPIPARMASK_CNT_U32  BitMaskRealWorld=Stored Integer
  Compare To Zero1 : simulink/Logic and Bit Operations/Compare To Zero  relop=>  OutDataTypeStr=boolean
  Compare To Zero2 : simulink/Logic and Bit Operations/Compare To Zero  relop===  OutDataTypeStr=boolean
  Constant : Constant  Value=SPIPARMASK_CNT_U32
  CopyRight2 : Subsystem  Description=|  mask(Copyright Information){none=on}
      | Copyright info block.                                               
      |                                                                     
      | Place copyright information at the top of every subsystem in design.
      mask prompts: none "No parameters"
      mask help: Place copyright information at the top of every subsystem in design.
      mask Display:
      | NxtrConf = 'Nexteer Confidential';
      | 
      | sys = bdroot; %handle for the current model ("system")
      | first = get_param(sys,'Created');
      | first = first(end-3:end);  %year is last four digits
      | 
      | last = get_param(sys,'LastModifiedDate');
      | if isempty(last)
      |     last = datestr(now,'yyyy');
      | else
      |     last = last(end-3:end);
      | end
      | 
      | if strcmp(first,last)
      |     fprintf('%s -- Copyright %s Nexteer',NxtrConf,first)
      | else
      |     fprintf('%s -- %s%s- %s Nexteer',NxtrConf,char(169),first,last)
      | end
  Sum : Sum  Inputs=|++
  MotAg1ParFlt : Outport
  wires:
  Bitwise Operator3/1 -> Compare To Zero1/1
  RxMtrPosReg_Cnt_u32/1 -> Bitwise Operator3/2, Compare To Zero2/1
  Compare To Zero1/1 -> Atomic Subsystem2/1(InputBoolean)
  Atomic Subsystem2/1(OutputNumber) -> Sum/1
  Compare To Zero2/1 -> Atomic Subsystem3/1(InputBoolean)
  Atomic Subsystem3/1(OutputNumber) -> Sum/2
  Sum/1 -> MotAg1ParFlt/1
  Constant/1 -> Bitwise Operator3/1

== system CM640A_MotAg1Meas/MotAg1Meas/MotAg1MeasPer1/Process MotAg1 Angle/Process MotAg1Raw/Raw Mecl Mot Ag Processing ==
  RxMtrPosReg_Cnt_u32 : Inport
  Constant : Constant  Value=SNSRAGMASK_CNT_U32
  CopyRight2 : Subsystem  Description=|  mask(Copyright Information){none=on}
      | Copyright info block.                                               
      |                                                                     
      | Place copyright information at the top of every subsystem in design.
      mask prompts: none "No parameters"
      mask help: Place copyright information at the top of every subsystem in design.
      mask Display:
      | NxtrConf = 'Nexteer Confidential';
      | 
      | sys = bdroot; %handle for the current model ("system")
      | first = get_param(sys,'Created');
      | first = first(end-3:end);  %year is last four digits
      | 
      | last = get_param(sys,'LastModifiedDate');
      | if isempty(last)
      |     last = datestr(now,'yyyy');
      | else
      |     last = last(end-3:end);
      | end
      | 
      | if strcmp(first,last)
      |     fprintf('%s -- Copyright %s Nexteer',NxtrConf,first)
      | else
      |     fprintf('%s -- %s%s- %s Nexteer',NxtrConf,char(169),first,last)
      | end
  Data Type Conversion2 : DataTypeConversion  OutDataTypeStr=uint16
  Input resolution - p13 : simulink/Logic and Bit Operations/Bitwise Operator  logicop=AND  UseBitMask=off  NumInputPorts=2  BitMask=SNSRAGMASK_CNT_U32  BitMaskRealWorld=Stored Integer
  Shift to p16 : ArithShift  BitShiftNumber=3  BitShiftDirection=Left
  MotAg1RawMecl : Outport
  wires:
  RxMtrPosReg_Cnt_u32/1 -> Input resolution - p13/1
  Input resolution - p13/1 -> Shift to p16/1
  Shift to p16/1 -> Data Type Conversion2/1
  Data Type Conversion2/1 -> MotAg1RawMecl/1
  Constant/1 -> Input resolution - p13/2

== system CM640A_MotAg1Meas/MotAg1Meas/MotAg1MeasPer1/Process MotAg1 Angle/Process MotAg1Raw/Undervoltage Bit Monitoring ==
  RxMtrPosReg_Cnt_u32 : Inport
  Atomic Subsystem1 : Subsystem  TreatAsAtomicUnit=on
  Bitwise Operator1 : simulink/Logic and Bit Operations/Bitwise Operator  logicop=AND  UseBitMask=off  NumInputPorts=2  BitMask=SNSRVLTGFLTMASK_CNT_U32  BitMaskRealWorld=Stored Integer
  Compare To Zero : simulink/Logic and Bit Operations/Compare To Zero  relop=>  OutDataTypeStr=boolean
  Constant : Constant  Value=SNSRVLTGFLTMASK_CNT_U32
  CopyRight2 : Subsystem  Description=|  mask(Copyright Information){none=on}
      | Copyright info block.                                               
      |                                                                     
      | Place copyright information at the top of every subsystem in design.
      mask prompts: none "No parameters"
      mask help: Place copyright information at the top of every subsystem in design.
      mask Display:
      | NxtrConf = 'Nexteer Confidential';
      | 
      | sys = bdroot; %handle for the current model ("system")
      | first = get_param(sys,'Created');
      | first = first(end-3:end);  %year is last four digits
      | 
      | last = get_param(sys,'LastModifiedDate');
      | if isempty(last)
      |     last = datestr(now,'yyyy');
      | else
      |     last = last(end-3:end);
      | end
      | 
      | if strcmp(first,last)
      |     fprintf('%s -- Copyright %s Nexteer',NxtrConf,first)
      | else
      |     fprintf('%s -- %s%s- %s Nexteer',NxtrConf,char(169),first,last)
      | end
  MotAg1VltgFlt : Outport
  wires:
  Compare To Zero/1 -> Atomic Subsystem1/1(InputBoolean)
  Bitwise Operator1/1 -> Compare To Zero/1
  RxMtrPosReg_Cnt_u32/1 -> Bitwise Operator1/1
  Atomic Subsystem1/1(OutputNumber) -> MotAg1VltgFlt/1
  Constant/1 -> Bitwise Operator1/2

== system CM640A_MotAg1Meas/MotAg1Meas/MotAg1MeasPer1/Process MotAg1 Angle/Protocol Present Handling/CopyRight2 ==

== system CM640A_MotAg1Meas/MotAg1Meas/MotAg1MeasPer1/Process MotAg1 Angle/Protocol Present Handling/Invalid Polarity, Hold Last Value ==
  In1 : Inport
  Action Port : ActionPort  ActionType=else
  Out1 : Outport
  wires:
  In1/1 -> Out1/1

== system CM640A_MotAg1Meas/MotAg1Meas/MotAg1MeasPer1/Process MotAg1 Angle/Protocol Present Handling/Valid Polarity ==
  In1 : Inport
  Action Port : ActionPort  ActionType=then
  Out1 : Outport
  wires:
  In1/1 -> Out1/1

== system CM640A_MotAg1Meas/MotAg1Meas/MotAg1MeasPer2/MotAg1 Protocol Fault Operation/Atomic Subsystem/CopyRight2 ==

== system CM640A_MotAg1Meas/MotAg1Meas/MotAg1MeasPer2/MotAg1 Protocol Fault Operation/Atomic Subsystem/N Step ==
  Action Port : ActionPort  ActionType=else
  Constant3 : Constant  Value=MOTAG1PRTCLFLTPASSSTEP_CNT_U16
  CopyRight2 : Subsystem  Description=|  mask(Copyright Information){none=on}
      | Copyright info block.                                               
      |                                                                     
      | Place copyright information at the top of every subsystem in design.
      mask prompts: none "No parameters"
      mask help: Place copyright information at the top of every subsystem in design.
      mask Display:
      | NxtrConf = 'Nexteer Confidential';
      | 
      | sys = bdroot; %handle for the current model ("system")
      | first = get_param(sys,'Created');
      | first = first(end-3:end);  %year is last four digits
      | 
      | last = get_param(sys,'LastModifiedDate');
      | if isempty(last)
      |     last = datestr(now,'yyyy');
      | else
      |     last = last(end-3:end);
      | end
      | 
      | if strcmp(first,last)
      |     fprintf('%s -- Copyright %s Nexteer',NxtrConf,first)
      | else
      |     fprintf('%s -- %s%s- %s Nexteer',NxtrConf,char(169),first,last)
      | end
  NtcNr1 : simulink/Sources/Enumerated Constant  OutDataTypeStr=Enum: NtcSts1  Value=NtcSts1.NTCSTS_PREPASSD  SampleTime=inf
  NtcSts : Outport
  DebStep : Outport  Port=2
  wires:
  Constant3/1 -> DebStep/1
  NtcNr1/1 -> NtcSts/1

== system CM640A_MotAg1Meas/MotAg1Meas/MotAg1MeasPer2/MotAg1 Protocol Fault Operation/Atomic Subsystem/P Step ==
  Action Port : ActionPort  ActionType=then
  Constant3 : Constant  Value=MOTAG1PRTCLFLTFAILSTEP_CNT_U16
  CopyRight2 : Subsystem  Description=|  mask(Copyright Information){none=on}
      | Copyright info block.                                               
      |                                                                     
      | Place copyright information at the top of every subsystem in design.
      mask prompts: none "No parameters"
      mask help: Place copyright information at the top of every subsystem in design.
      mask Display:
      | NxtrConf = 'Nexteer Confidential';
      | 
      | sys = bdroot; %handle for the current model ("system")
      | first = get_param(sys,'Created');
      | first = first(end-3:end);  %year is last four digits
      | 
      | last = get_param(sys,'LastModifiedDate');
      | if isempty(last)
      |     last = datestr(now,'yyyy');
      | else
      |     last = last(end-3:end);
      | end
      | 
      | if strcmp(first,last)
      |     fprintf('%s -- Copyright %s Nexteer',NxtrConf,first)
      | else
      |     fprintf('%s -- %s%s- %s Nexteer',NxtrConf,char(169),first,last)
      | end
  NtcNr1 : simulink/Sources/Enumerated Constant  OutDataTypeStr=Enum: NtcSts1  Value=NtcSts1.NTCSTS_PREFAILD  SampleTime=inf
  NtcSts : Outport
  DebStep : Outport  Port=2
  wires:
  NtcNr1/1 -> NtcSts/1
  Constant3/1 -> DebStep/1

== system CM640A_MotAg1Meas/MotAg1Meas/MotAg1MeasPer2/MotAg1 Protocol Fault Operation/GetNtcQlfr/CopyRight2 ==

== system CM640A_MotAg1Meas/MotAg1Meas/MotAg1MeasPer2/MotAg1 Protocol Fault Operation/SetNtcSts/CopyRight2 ==

== system CM640A_MotAg1Meas/MotAg1Meas/MotAg1MeasPer2/MotAg1 Protocol Fault Operation/Subsystem/Atomic Subsystem1 ==
  InputBoolean : Inport  OutDataTypeStr=boolean
  If : If  IfExpression=u1 ~= 0
  Merge : Merge
  Output 0 : Subsystem  TreatAsAtomicUnit=on
  Output 1 : Subsystem  TreatAsAtomicUnit=on
  OutputNumber : Outport  OutDataTypeStr=uint8
  wires:
  InputBoolean/1 -> If/1
  If/1 -> Output 1/Action
  If/2 -> Output 0/Action
  Output 1/1(Out1) -> Merge/1
  Output 0/1(Out1) -> Merge/2
  Merge/1 -> OutputNumber/1

== system CM640A_MotAg1Meas/MotAg1Meas/MotAg1MeasPer2/MotAg1 Protocol Fault Operation/Subsystem/Atomic Subsystem2 ==
  InputBoolean : Inport  OutDataTypeStr=boolean
  If : If  IfExpression=u1 ~= 0
  Merge : Merge
  Output 0 : Subsystem  TreatAsAtomicUnit=on
  Output 1 : Subsystem  TreatAsAtomicUnit=on
  OutputNumber : Outport  OutDataTypeStr=uint8
  wires:
  Merge/1 -> OutputNumber/1
  Output 0/1(Out1) -> Merge/2
  Output 1/1(Out1) -> Merge/1
  If/2 -> Output 0/Action
  If/1 -> Output 1/Action
  InputBoolean/1 -> If/1

== system CM640A_MotAg1Meas/MotAg1Meas/MotAg1MeasPer2/MotAg1 Protocol Fault Operation/Subsystem/Atomic Subsystem3 ==
  InputBoolean : Inport  OutDataTypeStr=boolean
  If : If  IfExpression=u1 ~= 0
  Merge : Merge
  Output 0 : Subsystem  TreatAsAtomicUnit=on
  Output 1 : Subsystem  TreatAsAtomicUnit=on
  OutputNumber : Outport  OutDataTypeStr=uint8
  wires:
  InputBoolean/1 -> If/1
  If/1 -> Output 1/Action
  If/2 -> Output 0/Action
  Output 1/1(Out1) -> Merge/1
  Output 0/1(Out1) -> Merge/2
  Merge/1 -> OutputNumber/1

== system CM640A_MotAg1Meas/MotAg1Meas/MotAg1MeasPer2/MotAg1 Protocol Fault Operation/Subsystem/CopyRight2 ==

== system CM640A_MotAg1Meas/MotAg1Meas/MotAg1MeasPer2/Process ErrorReg and DieRevCtr/Process MotAg1RawErr/CopyRight2 ==

== system CM640A_MotAg1Meas/MotAg1Meas/MotAg1MeasPer2/Process ErrorReg and DieRevCtr/Process MotAg1RawErr/Invalid Polarity, Hold Last Value ==
  In1 : Inport
  Action Port : ActionPort  ActionType=else
  CopyRight2 : Subsystem  Description=|  mask(Copyright Information){none=on}
      | Copyright info block.                                               
      |                                                                     
      | Place copyright information at the top of every subsystem in design.
      mask prompts: none "No parameters"
      mask help: Place copyright information at the top of every subsystem in design.
      mask Display:
      | NxtrConf = 'Nexteer Confidential';
      | 
      | sys = bdroot; %handle for the current model ("system")
      | first = get_param(sys,'Created');
      | first = first(end-3:end);  %year is last four digits
      | 
      | last = get_param(sys,'LastModifiedDate');
      | if isempty(last)
      |     last = datestr(now,'yyyy');
      | else
      |     last = last(end-3:end);
      | end
      | 
      | if strcmp(first,last)
      |     fprintf('%s -- Copyright %s Nexteer',NxtrConf,first)
      | else
      |     fprintf('%s -- %s%s- %s Nexteer',NxtrConf,char(169),first,last)
      | end
  Out1 : Outport  OutDataTypeStr=uint8
  wires:
  In1/1 -> Out1/1

== system CM640A_MotAg1Meas/MotAg1Meas/MotAg1MeasPer2/Process ErrorReg and DieRevCtr/Process MotAg1RawErr/Process MotAg1RawErr ==
  MotAg1ErrReg : Inport  OutDataTypeStr=uint32
  Atomic Subsystem1 : Subsystem  TreatAsAtomicUnit=on
  Atomic Subsystem2 : Subsystem  TreatAsAtomicUnit=on
  Bitwise Operator2 : simulink/Logic and Bit Operations/Bitwise Operator  logicop=AND  UseBitMask=off  NumInputPorts=2  BitMask=SNSRERRMASK_CNT_U32  BitMaskRealWorld=Stored Integer
  Bitwise Operator3 : simulink/Logic and Bit Operations/Bitwise Operator  logicop=AND  UseBitMask=off  NumInputPorts=2  BitMask=SPIPARMASK_CNT_U32  BitMaskRealWorld=Stored Integer
  Compare To Zero1 : simulink/Logic and Bit Operations/Compare To Zero  relop=>  OutDataTypeStr=boolean
  Compare To Zero2 : simulink/Logic and Bit Operations/Compare To Zero  relop===  OutDataTypeStr=boolean
  Constant : Constant  Value=SNSRERRMASK_CNT_U32
  Constant1 : Constant  Value=SPIPARMASK_CNT_U32
  CopyRight2 : Subsystem  Description=|  mask(Copyright Information){none=on}
      | Copyright info block.                                               
      |                                                                     
      | Place copyright information at the top of every subsystem in design.
      mask prompts: none "No parameters"
      mask help: Place copyright information at the top of every subsystem in design.
      mask Display:
      | NxtrConf = 'Nexteer Confidential';
      | 
      | sys = bdroot; %handle for the current model ("system")
      | first = get_param(sys,'Created');
      | first = first(end-3:end);  %year is last four digits
      | 
      | last = get_param(sys,'LastModifiedDate');
      | if isempty(last)
      |     last = datestr(now,'yyyy');
      | else
      |     last = last(end-3:end);
      | end
      | 
      | if strcmp(first,last)
      |     fprintf('%s -- Copyright %s Nexteer',NxtrConf,first)
      | else
      |     fprintf('%s -- %s%s- %s Nexteer',NxtrConf,char(169),first,last)
      | end
  Data Type Conversion2 : DataTypeConversion  OutDataTypeStr=uint8
  Sum : Sum  Inputs=|++
  MotAg1ErrParFlt : Outport
  MotAg1Err : Outport  Port=2
  wires:
  Bitwise Operator3/1 -> Compare To Zero1/1
  MotAg1ErrReg/1 -> Bitwise Operator2/1, Bitwise Operator3/2, Compare To Zero2/1
  Data Type Conversion2/1 -> MotAg1Err/1
  Bitwise Operator2/1 -> Data Type Conversion2/1
  Compare To Zero1/1 -> Atomic Subsystem1/1(InputBoolean)
  Compare To Zero2/1 -> Atomic Subsystem2/1(InputBoolean)
  Atomic Subsystem2/1(OutputNumber) -> Sum/2
  Atomic Subsystem1/1(OutputNumber) -> Sum/1
  Sum/1 -> MotAg1ErrParFlt/1
  Constant/1 -> Bitwise Operator2/2
  Constant1/1 -> Bitwise Operator3/1

== system CM640A_MotAg1Meas/MotAg1Meas/MotAg1MeasPer2/Process ErrorReg and DieRevCtr/Process MotAg1RawErr/Valid Polarity ==
  In1 : Inport
  Action Port : ActionPort  ActionType=then
  CopyRight2 : Subsystem  Description=|  mask(Copyright Information){none=on}
      | Copyright info block.                                               
      |                                                                     
      | Place copyright information at the top of every subsystem in design.
      mask prompts: none "No parameters"
      mask help: Place copyright information at the top of every subsystem in design.
      mask Display:
      | NxtrConf = 'Nexteer Confidential';
      | 
      | sys = bdroot; %handle for the current model ("system")
      | first = get_param(sys,'Created');
      | first = first(end-3:end);  %year is last four digits
      | 
      | last = get_param(sys,'LastModifiedDate');
      | if isempty(last)
      |     last = datestr(now,'yyyy');
      | else
      |     last = last(end-3:end);
      | end
      | 
      | if strcmp(first,last)
      |     fprintf('%s -- Copyright %s Nexteer',NxtrConf,first)
      | else
      |     fprintf('%s -- %s%s- %s Nexteer',NxtrConf,char(169),first,last)
      | end
  Out1 : Outport  OutDataTypeStr=uint8
  wires:
  In1/1 -> Out1/1

== system CM640A_MotAg1Meas/MotAg1Meas/MotAg1MeasInit1/Compute Correction Table/NVM NOK/Zero out correction table/CopyRight2 ==
